simulink model "Droop_Control_MG_4DGs"  (R2024a)
settings: Solver=ode3  StartTime=0.0  StopTime=10  FixedStep=2e-5  RelTol=1e-3  EnableMultiTasking=on
InitFcn:
  | Kp_V = 4;
  | Ki_V = 800;
  | Kp_I = 5;
  | Ki_I = 110;
values from neighbouring files (symbols this model uses):
  DG = cell(1, numOfDGs)    [evaluateDesigns.m]
  Line = cell(1, numOfLines)    [evaluateDesigns.m]
  numOfDGs = size(B_il,1)    [OptimizeMGparameters.m]    (also in OptimizepValsMethod1.m; centralizedCodesign.m; centralizedCodesignFeasibility.m; centralizedLocalControlDesign-Mohammad’s Laptop.m)
  V_ref = 48    [Global_Controller_Synthesis.m]
undefined symbols (not defined in the file or in its folder): PlugIn, PlugOut, V_nom
libraries: spsSeriesRLCBranchLib x28, spsCurrentMeasurementLib x8, spsVoltageMeasurementLib x5, spsIdealSwitchLib x4, spsStairGeneratorLib x4, spsControlledCurrentSourceLib x4, spsDCVoltageSourceLib x4, spsDiodeLib x4, spsIGBTLib x4, simulink x4, spspowerguiLib x1
settings Model: Creator=Guo Fanghong Admin  LastModifiedBy=najaf
settings SolverCC: AlgebraicLoopSolver=TrustRegion
settings DataIOCC: LimitDataPoints=on  SaveFormat=Array  SignalLoggingSaveFormat=ModelDataLogs
settings OptimizationCC: ExpressionDepthLimit=2147483647  LifeSpan=inf
settings DebuggingCC: UnderspecifiedInitializationDetection=Classic  MergeDetectMultiDrivingBlocksExec=none  SolverPrmCheckMsg=warning  FcnCallInpInsideContextMsg=warning  UnconnectedInputMsg=warning  UnconnectedOutputMsg=warning  UnconnectedLineMsg=warning  StateNameClashWarn=warning  SFUnexpectedBacktrackingDiag=warning  SFNoUnconditionalDefaultTransitionDiag=warning  SFExecutionAtInitializationDiag=none  ArithmeticOperatorsInVariantConditions=warning
settings HardwareCC: ProdBitPerPointer=32  ProdBitPerSizeT=32  ProdBitPerPtrDiffT=32  ProdLargestAtomicFloat=None  ProdIntDivRoundTo=Undefined  ProdEndianess=Unspecified  ProdWordSize=32  ProdHWDeviceType=32-bit Generic
settings ModelReferenceCC: EnableRefExpFcnMdlSchedulingChecks=on  PropagateSignalLabelsOutOfModel=off
settings SFSimCC: SimUseLocalCustomCode=off  CustomCodeUndefinedFunction=UseInterfaceOnly
settings RTWCC: RTWUseLocalCustomCode=off  GPUComputeCapability=3.5
settings CodeAppCC: StateflowObjectComments=on
settings GRTTargetCC: TargetLangStandard=C89/C90 (ANSI)
settings ConfigComp: CovMetricSettings=dw  CovSaveCumulativeToWorkspaceVar=on  CovSaveSingleToWorkspaceVar=on  CovExternalEMLEnable=off  CovSFcnEnable=off
settings SimscapeCC: SimscapeNormalizeSystem=off

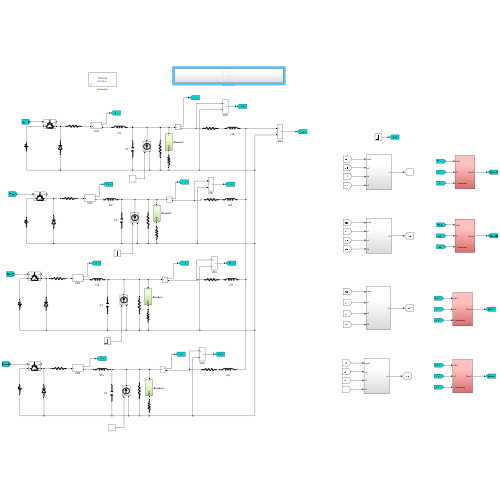
[thumbnail: Simulink's stored preview of the top-level diagram]
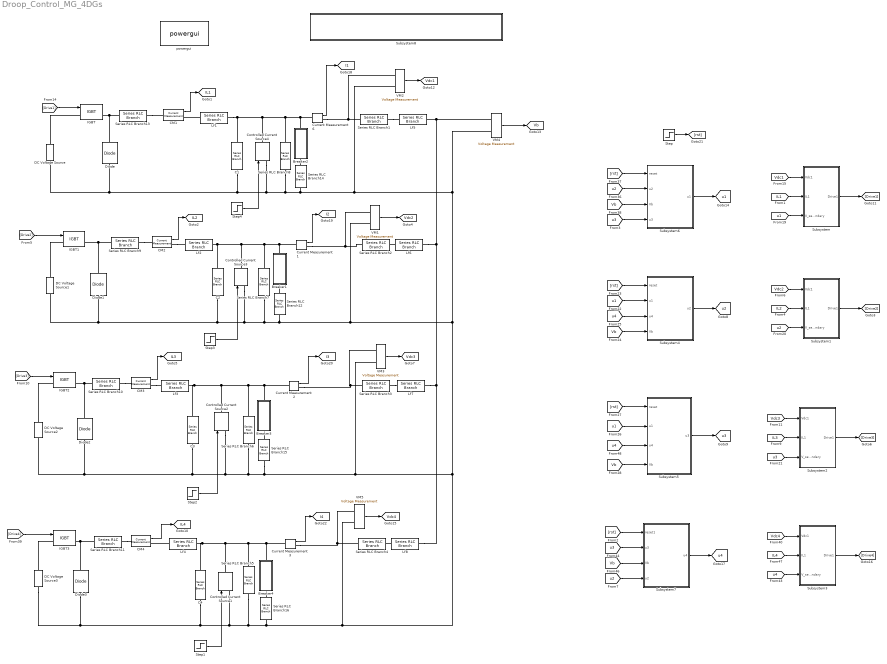
== system Droop_Control_MG_4DGs ==
  Breaker1 : Subsystem
  Breaker2 : Subsystem
  Breaker3 : Subsystem
  Breaker4 : Subsystem
  C1 : spsSeriesRLCBranchLib/Series RLC Branch  LConnTagsString=__new0  RConnTagsString=__new0  BranchType=C  Resistance=0  Inductance=0  SetiL0=off  InitialCurrent=0  Capacitance=DG{1}.C  Setx0=off  InitialVoltage=0  Measurements=None
  C2 : spsSeriesRLCBranchLib/Series RLC Branch  LConnTagsString=__new0  RConnTagsString=__new0  BranchType=C  Resistance=0  Inductance=0  SetiL0=off  InitialCurrent=0  Capacitance=DG{2}.C  Setx0=off  InitialVoltage=0  Measurements=None
  C3 : spsSeriesRLCBranchLib/Series RLC Branch  LConnTagsString=__new0  RConnTagsString=__new0  BranchType=C  Resistance=0  Inductance=0  SetiL0=off  InitialCurrent=0  Capacitance=DG{3}.C  Setx0=off  InitialVoltage=0  Measurements=None
  C4 : spsSeriesRLCBranchLib/Series RLC Branch  LConnTagsString=__new0  RConnTagsString=__new0  BranchType=C  Resistance=0  Inductance=0  SetiL0=off  InitialCurrent=0  Capacitance=DG{4}.C  Setx0=off  InitialVoltage=0  Measurements=None
  CM{1..4} (4 alike) : spsCurrentMeasurementLib/Current Measurement  PhasorSimulation=off  OutputType=Complex  PSBequivalent=0
  Controlled Current Source1 : spsControlledCurrentSourceLib/Controlled Current Source  Initialize=on  Source_Type=DC  Amplitude=5*DG{4}.IL  Phase=0  Frequency=0  Measurements=None
  Controlled Current Source2 : spsControlledCurrentSourceLib/Controlled Current Source  Initialize=on  Source_Type=DC  Amplitude=5*DG{3}.IL  Phase=0  Frequency=0  Measurements=None
  Controlled Current Source3 : spsControlledCurrentSourceLib/Controlled Current Source  Initialize=on  Source_Type=DC  Amplitude=5*DG{2}.IL  Phase=0  Frequency=0  Measurements=None
  Controlled Current Source4 : spsControlledCurrentSourceLib/Controlled Current Source  Initialize=on  Source_Type=DC  Amplitude=5*DG{1}.IL  Phase=0  Frequency=0  Measurements=None
  Current Measurement{1..3,6} (4 alike) : spsCurrentMeasurementLib/Current Measurement  PhasorSimulation=off  OutputType=Complex  PSBequivalent=0
  DC Voltage Source{,1..3} (4 alike) : spsDCVoltageSourceLib/DC Voltage Source  Amplitude=V_nom  Measurements=None
  Diode{,1..3} (4 alike) : spsDiodeLib/Diode  Ron=0.001  Lon=0  Vf=0.8  IC=0  UseSnubber=off  Rs=500  Cs=0  Measurements=off
  IGBT{,1..3} (4 alike) : spsIGBTLib/IGBT  Ron=0.001  Lon=0  Vf=1  Tf=1e-6  Tt=2e-6  IC=0  Rs=1e5  Cs=inf  Measurements=on
  Lf1 : spsSeriesRLCBranchLib/Series RLC Branch  LConnTagsString=__new0  RConnTagsString=__new0  BranchType=L  Resistance=0  Inductance=DG{1}.L  SetiL0=off  InitialCurrent=0  Capacitance=inf  Setx0=off  InitialVoltage=0  Measurements=Branch current
  Lf2 : spsSeriesRLCBranchLib/Series RLC Branch  LConnTagsString=__new0  RConnTagsString=__new0  BranchType=L  Resistance=0  Inductance=DG{2}.L  SetiL0=off  InitialCurrent=0  Capacitance=inf  Setx0=off  InitialVoltage=0  Measurements=Branch current
  Lf3 : spsSeriesRLCBranchLib/Series RLC Branch  LConnTagsString=__new0  RConnTagsString=__new0  BranchType=L  Resistance=0  Inductance=DG{3}.L  SetiL0=off  InitialCurrent=0  Capacitance=inf  Setx0=off  InitialVoltage=0  Measurements=Branch current
  Lf4 : spsSeriesRLCBranchLib/Series RLC Branch  LConnTagsString=__new0  RConnTagsString=__new0  BranchType=L  Resistance=0  Inductance=DG{4}.L  SetiL0=off  InitialCurrent=0  Capacitance=inf  Setx0=off  InitialVoltage=0  Measurements=Branch current
  Lf5 : spsSeriesRLCBranchLib/Series RLC Branch  LConnTagsString=__new0  RConnTagsString=__new0  BranchType=L  Resistance=0  Inductance=Line{1}.L  SetiL0=off  InitialCurrent=0  Capacitance=inf  Setx0=off  InitialVoltage=0  Measurements=Branch current
  Lf6 : spsSeriesRLCBranchLib/Series RLC Branch  LConnTagsString=__new0  RConnTagsString=__new0  BranchType=L  Resistance=0  Inductance=Line{2}.L  SetiL0=off  InitialCurrent=0  Capacitance=inf  Setx0=off  InitialVoltage=0  Measurements=Branch current
  Lf7 : spsSeriesRLCBranchLib/Series RLC Branch  LConnTagsString=__new0  RConnTagsString=__new0  BranchType=L  Resistance=0  Inductance=Line{3}.L  SetiL0=off  InitialCurrent=0  Capacitance=inf  Setx0=off  InitialVoltage=0  Measurements=Branch current
  Lf8 : spsSeriesRLCBranchLib/Series RLC Branch  LConnTagsString=__new0  RConnTagsString=__new0  BranchType=L  Resistance=0  Inductance=Line{4}.L  SetiL0=off  InitialCurrent=0  Capacitance=inf  Setx0=off  InitialVoltage=0  Measurements=Branch current
  Series RLC Branch1 : spsSeriesRLCBranchLib/Series RLC Branch  LConnTagsString=__new0  RConnTagsString=__new0  BranchType=R  Resistance=Line{1}.R  Inductance=0.25154  SetiL0=off  InitialCurrent=0  Capacitance=1e-6  Setx0=off  InitialVoltage=0  Measurements=None
  Series RLC Branch10 : spsSeriesRLCBranchLib/Series RLC Branch  LConnTagsString=__new0  RConnTagsString=__new0  BranchType=R  Resistance=DG{3}.R  Inductance=0.25154  SetiL0=off  InitialCurrent=0  Capacitance=1e-6  Setx0=off  InitialVoltage=0  Measurements=None
  Series RLC Branch11 : spsSeriesRLCBranchLib/Series RLC Branch  LConnTagsString=__new0  RConnTagsString=__new0  BranchType=R  Resistance=DG{4}.R  Inductance=0.25154  SetiL0=off  InitialCurrent=0  Capacitance=1e-6  Setx0=off  InitialVoltage=0  Measurements=None
  Series RLC Branch12 : spsSeriesRLCBranchLib/Series RLC Branch  LConnTagsString=__new0  RConnTagsString=__new0  BranchType=R  Resistance=0.5*DG{2}.Y  Inductance=1e-2  SetiL0=off  InitialCurrent=0  Capacitance=2.2e-3  Setx0=off  InitialVoltage=0  Measurements=None
  Series RLC Branch13 : spsSeriesRLCBranchLib/Series RLC Branch  LConnTagsString=__new0  RConnTagsString=__new0  BranchType=R  Resistance=DG{1}.R  Inductance=0.25154  SetiL0=off  InitialCurrent=0  Capacitance=1e-6  Setx0=off  InitialVoltage=0  Measurements=None
  Series RLC Branch14 : spsSeriesRLCBranchLib/Series RLC Branch  LConnTagsString=__new0  RConnTagsString=__new0  BranchType=R  Resistance=0.5*DG{1}.Y  Inductance=1e-2  SetiL0=off  InitialCurrent=0  Capacitance=2.2e-3  Setx0=off  InitialVoltage=0  Measurements=None
  Series RLC Branch15 : spsSeriesRLCBranchLib/Series RLC Branch  LConnTagsString=__new0  RConnTagsString=__new0  BranchType=R  Resistance=0.5*DG{3}.Y  Inductance=1e-2  SetiL0=off  InitialCurrent=0  Capacitance=2.2e-3  Setx0=off  InitialVoltage=0  Measurements=None
  Series RLC Branch16 : spsSeriesRLCBranchLib/Series RLC Branch  LConnTagsString=__new0  RConnTagsString=__new0  BranchType=R  Resistance=0.5*DG{4}.Y  Inductance=1e-2  SetiL0=off  InitialCurrent=0  Capacitance=2.2e-3  Setx0=off  InitialVoltage=0  Measurements=None
  Series RLC Branch2 : spsSeriesRLCBranchLib/Series RLC Branch  LConnTagsString=__new0  RConnTagsString=__new0  BranchType=R  Resistance=Line{2}.R  Inductance=0.25154  SetiL0=off  InitialCurrent=0  Capacitance=1e-6  Setx0=off  InitialVoltage=0  Measurements=None
  Series RLC Branch3 : spsSeriesRLCBranchLib/Series RLC Branch  LConnTagsString=__new0  RConnTagsString=__new0  BranchType=R  Resistance=Line{3}.R  Inductance=0.25154  SetiL0=off  InitialCurrent=0  Capacitance=1e-6  Setx0=off  InitialVoltage=0  Measurements=None
  Series RLC Branch4 : spsSeriesRLCBranchLib/Series RLC Branch  LConnTagsString=__new0  RConnTagsString=__new0  BranchType=R  Resistance=Line{4}.R  Inductance=0.25154  SetiL0=off  InitialCurrent=0  Capacitance=1e-6  Setx0=off  InitialVoltage=0  Measurements=None
  Series RLC Branch5 : spsSeriesRLCBranchLib/Series RLC Branch  LConnTagsString=__new0  RConnTagsString=__new0  BranchType=R  Resistance=DG{4}.Y  Inductance=0.25154  SetiL0=off  InitialCurrent=0  Capacitance=1e-6  Setx0=off  InitialVoltage=0  Measurements=None
  Series RLC Branch6 : spsSeriesRLCBranchLib/Series RLC Branch  LConnTagsString=__new0  RConnTagsString=__new0  BranchType=R  Resistance=DG{3}.Y  Inductance=0.25154  SetiL0=off  InitialCurrent=0  Capacitance=1e-6  Setx0=off  InitialVoltage=0  Measurements=None
  Series RLC Branch7 : spsSeriesRLCBranchLib/Series RLC Branch  LConnTagsString=__new0  RConnTagsString=__new0  BranchType=R  Resistance=DG{2}.Y  Inductance=0.25154  SetiL0=off  InitialCurrent=0  Capacitance=1e-6  Setx0=off  InitialVoltage=0  Measurements=None
  Series RLC Branch8 : spsSeriesRLCBranchLib/Series RLC Branch  LConnTagsString=__new0  RConnTagsString=__new0  BranchType=R  Resistance=DG{1}.Y  Inductance=0.25154  SetiL0=off  InitialCurrent=0  Capacitance=1e-6  Setx0=off  InitialVoltage=0  Measurements=None
  Series RLC Branch9 : spsSeriesRLCBranchLib/Series RLC Branch  LConnTagsString=__new0  RConnTagsString=__new0  BranchType=R  Resistance=DG{2}.R  Inductance=0.25154  SetiL0=off  InitialCurrent=0  Capacitance=1e-6  Setx0=off  InitialVoltage=0  Measurements=None
  Step : Step  SampleTime=0
  Step{1..4} (4 alike) : Step  Time=3  SampleTime=0
  Subsystem : Subsystem
  Subsystem1 : Subsystem
  Subsystem2 : Subsystem
  Subsystem3 : Subsystem
  Subsystem4 : Subsystem
  Subsystem5 : Subsystem
  Subsystem6 : Subsystem
  Subsystem7 : Subsystem
  Subsystem8 : Subsystem
  VM{1..5} (5 alike) : spsVoltageMeasurementLib/Voltage Measurement  PhasorSimulation=off  OutputType=Complex  PSBequivalent=0
  powergui : spspowerguiLib/powergui  Priority=1  SimulationMode=Discrete  SampleTime=2e-5  frequency=60  Iterations=50  frequencyindice=0  Pbase=100e6  ErrMax=1e-4  UnitsV=kV  UnitsW=MW  buscounter=0  FunctionMessages=off  echomessages=off  EnableUseOfTLC=off  CurrentSourceSwitches=off  DisableSnubberDevices=off  DisableRonSwitches=off  DisableVfSwitches=off  DisplayEquations=off  AutomaticDiscreteSolvers=off  SolverType=Tustin  Interpol=off  ExternalGateDelay=off  methode=off  Ts=0  x0status=steady  SPID=off  SwTol=0  HookPort=off  NonlinearTolerance=1e-4  nMaxIteration=100  ContinueOnMaxIteration=off  RestoreLinks=warning  ResistiveCurrentMeasurement=off  Frange=[0:2:500]  Ylog=off  Xlog=on  ShowGrid=off  save=off  variable=ZData  structure=0  ZoomFFT=off  StartTime=0.0  cycles=1  DisplayStyle=1  fundamental=60  FreqAxis=off  MaxFrequency=1000  frequencyindicesteady=1  RmsSteady=1  display=off
  tag scope: I1=global, I2=global, I3=global, I4=global, IL1=global, IL2=global, IL3=global, IL4=global, Vb=global, Vdc1=global, Vdc2=global, Vdc3=global, Vdc4=global, u1=global, u2=global, u3=global, u4=global
  wires:
  [Drive1] -> IGBT/1
  VM2/1 -> [Vdc1]
  CM1/1 -> [IL1]
  Subsystem/1(Drive1) -> [Drive1]
  [Vdc1] -> Subsystem/1(Vdc1)
  [IL1] -> Subsystem/2(IL1)
  [u1] -> Subsystem/3(V_secondary)
  [Drive2] -> IGBT1/1
  VM1/1 -> [Vdc2]
  CM2/1 -> [IL2]
  Subsystem1/1(Drive1) -> [Drive2]
  [Vdc2] -> Subsystem1/1(Vdc1)
  [IL2] -> Subsystem1/2(IL1)
  [u2] -> Subsystem1/3(V_secondary)
  [Drive3] -> IGBT2/1
  VM3/1 -> [Vdc3]
  CM3/1 -> [IL3]
  Subsystem2/1(Drive1) -> [Drive3]
  [Vdc3] -> Subsystem2/1(Vdc1)
  [IL3] -> Subsystem2/2(IL1)
  [u3] -> Subsystem2/3(V_secondary)
  Step/1 -> [rst]
  [u2] -> Subsystem6/2(u2)
  [rst] -> Subsystem6/1(reset)
  [Vb] -> Subsystem6/3(Vb)
  Subsystem6/1(u1) -> [u1]
  [u1] -> Subsystem4/2(u1)
  [rst] -> Subsystem4/1(reset)
  [Vb] -> Subsystem4/4(Vb)
  [u4] -> Subsystem4/3(u4)
  Subsystem4/1(u2) -> [u2]
  [u1] -> Subsystem5/2(u1)
  [rst] -> Subsystem5/1(reset)
  [Vb] -> Subsystem5/4(Vb)
  Subsystem5/1(u3) -> [u3]
  [Drive4] -> IGBT3/1
  VM5/1 -> [Vdc4]
  CM4/1 -> [IL4]
  Subsystem3/1(Drive1) -> [Drive4]
  [Vdc4] -> Subsystem3/1(Vdc1)
  [IL4] -> Subsystem3/2(IL1)
  [u4] -> Subsystem3/3(V_secondary)
  [u3] -> Subsystem7/2(u3)
  [rst] -> Subsystem7/1(reset1)
  [Vb] -> Subsystem7/3(Vb)
  Subsystem7/1(u4) -> [u4]
  [u4] -> Subsystem5/3(u4)
  VM4/1 -> [Vb]
  Step1/1 -> Controlled Current Source1/1
  Step2/1 -> Controlled Current Source2/1
  Step3/1 -> Controlled Current Source3/1
  Step4/1 -> Controlled Current Source4/1
  Current Measurement6/1 -> [I1]
  Current Measurement1/1 -> [I2]
  Current Measurement2/1 -> [I3]
  Current Measurement3/1 -> [I4]
  [u3] -> Subsystem6/4(u3)
  [u2] -> Subsystem7/4(u2)
  connections:
  C2/RConn1 -- Controlled Current Source3/LConn1 -- Series RLC Branch7/RConn1 -- Series RLC Branch12/RConn1 -- VM4/LConn2 -- VM2/LConn2 -- Series RLC Branch14/RConn1 -- Series RLC Branch8/RConn1 -- Controlled Current Source4/LConn1 -- C1/RConn1 -- Diode/LConn1 -- DC Voltage Source/LConn1 -- Controlled Current Source1/LConn1 -- Diode3/LConn1 -- DC Voltage Source3/LConn1 -- C4/RConn1 -- Series RLC Branch5/RConn1 -- Series RLC Branch16/RConn1 -- VM5/LConn2 -- Series RLC Branch15/RConn1 -- Series RLC Branch6/RConn1 -- Controlled Current Source2/LConn1 -- C3/RConn1 -- DC Voltage Source2/LConn1 -- Diode2/LConn1 -- VM3/LConn2 -- VM1/LConn2 -- Diode1/LConn1 -- DC Voltage Source1/LConn1
  Diode/RConn1 -- Series RLC Branch13/LConn1 -- IGBT/RConn1
  Lf1/RConn1 -- Current Measurement6/LConn1 -- Breaker2/RConn1 -- Series RLC Branch8/LConn1 -- Controlled Current Source4/RConn1 -- C1/LConn1
  IGBT/LConn1 -- DC Voltage Source/RConn1
  Diode1/RConn1 -- Series RLC Branch9/LConn1 -- IGBT1/RConn1
  IGBT1/LConn1 -- DC Voltage Source1/RConn1
  Series RLC Branch10/RConn1 -- CM3/LConn1
  IGBT2/LConn1 -- DC Voltage Source2/RConn1
  Series RLC Branch7/LConn1 -- Current Measurement1/LConn1 -- Breaker1/RConn1 -- Controlled Current Source3/RConn1 -- Lf2/RConn1 -- C2/LConn1
  Series RLC Branch6/LConn1 -- Current Measurement2/LConn1 -- Breaker3/RConn1 -- Controlled Current Source2/RConn1 -- Lf3/RConn1 -- C3/LConn1
  Lf8/RConn1 -- Lf7/RConn1 -- Lf6/RConn1 -- VM4/LConn1 -- Lf5/RConn1
  Series RLC Branch11/RConn1 -- CM4/LConn1
  Series RLC Branch4/LConn1 -- Current Measurement3/RConn1 -- VM5/LConn1
  IGBT3/LConn1 -- DC Voltage Source3/RConn1
  Lf1/LConn1 -- CM1/RConn1
  CM2/RConn1 -- Lf2/LConn1
  CM3/RConn1 -- Lf3/LConn1
  Lf4/LConn1 -- CM4/RConn1
  Series RLC Branch13/RConn1 -- CM1/LConn1
  Series RLC Branch9/RConn1 -- CM2/LConn1
  Diode2/RConn1 -- Series RLC Branch10/LConn1 -- IGBT2/RConn1
  Diode3/RConn1 -- Series RLC Branch11/LConn1 -- IGBT3/RConn1
  Series RLC Branch1/RConn1 -- Lf5/LConn1
  Series RLC Branch2/RConn1 -- Lf6/LConn1
  Series RLC Branch3/RConn1 -- Lf7/LConn1
  Series RLC Branch4/RConn1 -- Lf8/LConn1
  Series RLC Branch14/LConn1 -- Breaker2/LConn1
  Series RLC Branch12/LConn1 -- Breaker1/LConn1
  Series RLC Branch15/LConn1 -- Breaker3/LConn1
  Series RLC Branch16/LConn1 -- Breaker4/LConn1
  Series RLC Branch1/LConn1 -- VM2/LConn1 -- Current Measurement6/RConn1
  Series RLC Branch2/LConn1 -- Current Measurement1/RConn1 -- VM1/LConn1
  VM3/LConn1 -- Current Measurement2/RConn1 -- Series RLC Branch3/LConn1
  Controlled Current Source1/RConn1 -- Current Measurement3/LConn1 -- Breaker4/RConn1 -- Series RLC Branch5/LConn1 -- Lf4/RConn1 -- C4/LConn1

== system Droop_Control_MG_4DGs/Breaker1 ==
  Ideal Switch : spsIdealSwitchLib/Ideal Switch  Ron=0.001  Lon=0  IC=0  Rs=1e5  Cs=inf  Measurements=on
  Stair Generator : spsStairGeneratorLib/Stair Generator  t=[0,PlugOut,PlugIn]  e=[1, 0, 1]  Ts=0
  DG1 : PMIOPort  Side=Left
  + : PMIOPort  Port=2  Side=Right
  wires:
  Stair Generator/1 -> Ideal Switch/1
  connections:
  Ideal Switch/LConn1 -- DG1/RConn1
  Ideal Switch/RConn1 -- +/RConn1

== system Droop_Control_MG_4DGs/Breaker2 ==
  Ideal Switch : spsIdealSwitchLib/Ideal Switch  Ron=0.001  Lon=0  IC=0  Rs=1e5  Cs=inf  Measurements=on
  Stair Generator : spsStairGeneratorLib/Stair Generator  t=[0,PlugOut,PlugIn]  e=[1, 0, 1]  Ts=0
  DG1 : PMIOPort  Side=Left
  + : PMIOPort  Port=2  Side=Right
  wires:
  Stair Generator/1 -> Ideal Switch/1
  connections:
  Ideal Switch/RConn1 -- +/RConn1
  Ideal Switch/LConn1 -- DG1/RConn1

== system Droop_Control_MG_4DGs/Breaker3 ==
  Ideal Switch : spsIdealSwitchLib/Ideal Switch  Ron=0.001  Lon=0  IC=0  Rs=1e5  Cs=inf  Measurements=on
  Stair Generator : spsStairGeneratorLib/Stair Generator  t=[0,PlugOut,PlugIn]  e=[1, 0, 1]  Ts=0
  DG1 : PMIOPort  Side=Left
  + : PMIOPort  Port=2  Side=Right
  wires:
  Stair Generator/1 -> Ideal Switch/1
  connections:
  Ideal Switch/RConn1 -- +/RConn1
  Ideal Switch/LConn1 -- DG1/RConn1

== system Droop_Control_MG_4DGs/Breaker4 ==
  Ideal Switch : spsIdealSwitchLib/Ideal Switch  Ron=0.001  Lon=0  IC=0  Rs=1e5  Cs=inf  Measurements=on
  Stair Generator : spsStairGeneratorLib/Stair Generator  t=[0,PlugOut,PlugIn]  e=[1, 0, 1]  Ts=0
  DG1 : PMIOPort  Side=Left
  + : PMIOPort  Port=2  Side=Right
  wires:
  Stair Generator/1 -> Ideal Switch/1
  connections:
  Ideal Switch/LConn1 -- DG1/RConn1
  Ideal Switch/RConn1 -- +/RConn1

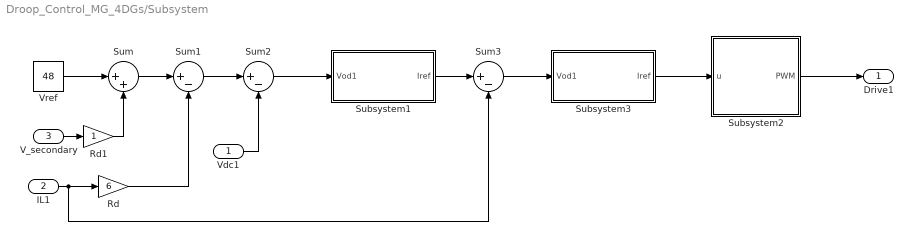
== system Droop_Control_MG_4DGs/Subsystem ==
  Vdc1 : Inport
  IL1 : Inport  Port=2
  V_secondary : Inport  Port=3
  Rd : Gain  Gain=6
  Rd1 : Gain
  Subsystem1 : Subsystem
      mask Display: disp('Voltage Controller')
  Subsystem2 : Subsystem
      mask Display: disp('PWM')
  Subsystem3 : Subsystem
      mask Display: disp('Current Controller')
  Sum : Sum  Inputs=|++
  Sum1 : Sum  Inputs=|+-
  Sum2 : Sum  Inputs=|+-
  Sum3 : Sum  Inputs=|+-
  Vref : Constant  Value=48
  Drive1 : Outport
  wires:
  Subsystem2/1(PWM) -> Drive1/1
  Vref/1 -> Sum/1
  Sum/1 -> Sum1/1
  V_secondary/1 -> Rd1/1
  Rd/1 -> Sum1/2
  IL1/1 -> Rd/1, Sum3/2
  Sum1/1 -> Sum2/1
  Vdc1/1 -> Sum2/2
  Sum2/1 -> Subsystem1/1(Vod1)
  Subsystem3/1(Iref) -> Subsystem2/1(u)
  Subsystem1/1(Iref) -> Sum3/1
  Sum3/1 -> Subsystem3/1(Vod1)
  Rd1/1 -> Sum/2

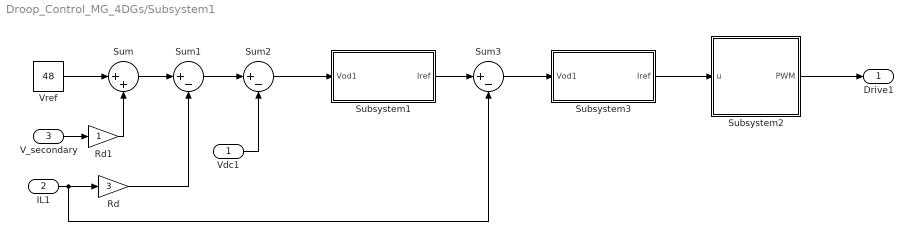
== system Droop_Control_MG_4DGs/Subsystem1 ==
  Vdc1 : Inport
  IL1 : Inport  Port=2
  V_secondary : Inport  Port=3
  Rd : Gain  Gain=3
  Rd1 : Gain
  Subsystem1 : Subsystem
      mask Display: disp('Voltage Controller')
  Subsystem2 : Subsystem
      mask Display: disp('PWM')
  Subsystem3 : Subsystem
      mask Display: disp('Current Controller')
  Sum : Sum  Inputs=|++
  Sum1 : Sum  Inputs=|+-
  Sum2 : Sum  Inputs=|+-
  Sum3 : Sum  Inputs=|+-
  Vref : Constant  Value=48
  Drive1 : Outport
  wires:
  Subsystem2/1(PWM) -> Drive1/1
  Vref/1 -> Sum/1
  Sum/1 -> Sum1/1
  V_secondary/1 -> Rd1/1
  Rd/1 -> Sum1/2
  IL1/1 -> Rd/1, Sum3/2
  Sum1/1 -> Sum2/1
  Vdc1/1 -> Sum2/2
  Sum2/1 -> Subsystem1/1(Vod1)
  Subsystem3/1(Iref) -> Subsystem2/1(u)
  Subsystem1/1(Iref) -> Sum3/1
  Sum3/1 -> Subsystem3/1(Vod1)
  Rd1/1 -> Sum/2

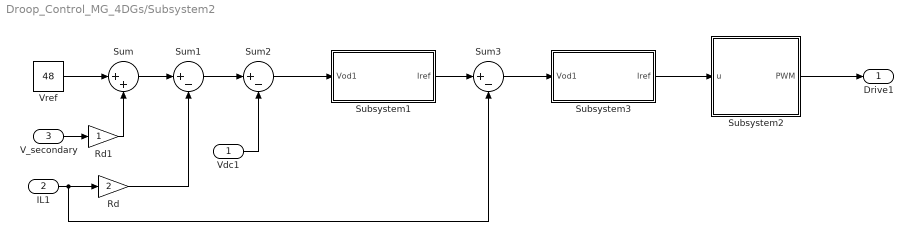
== system Droop_Control_MG_4DGs/Subsystem2 ==
  Vdc1 : Inport
  IL1 : Inport  Port=2
  V_secondary : Inport  Port=3
  Rd : Gain  Gain=2
  Rd1 : Gain
  Subsystem1 : Subsystem
      mask Display: disp('Voltage Controller')
  Subsystem2 : Subsystem
      mask Display: disp('PWM')
  Subsystem3 : Subsystem
      mask Display: disp('Current Controller')
  Sum : Sum  Inputs=|++
  Sum1 : Sum  Inputs=|+-
  Sum2 : Sum  Inputs=|+-
  Sum3 : Sum  Inputs=|+-
  Vref : Constant  Value=48
  Drive1 : Outport
  wires:
  Subsystem2/1(PWM) -> Drive1/1
  Vref/1 -> Sum/1
  Sum/1 -> Sum1/1
  V_secondary/1 -> Rd1/1
  Rd/1 -> Sum1/2
  IL1/1 -> Rd/1, Sum3/2
  Sum1/1 -> Sum2/1
  Vdc1/1 -> Sum2/2
  Sum2/1 -> Subsystem1/1(Vod1)
  Subsystem3/1(Iref) -> Subsystem2/1(u)
  Subsystem1/1(Iref) -> Sum3/1
  Sum3/1 -> Subsystem3/1(Vod1)
  Rd1/1 -> Sum/2

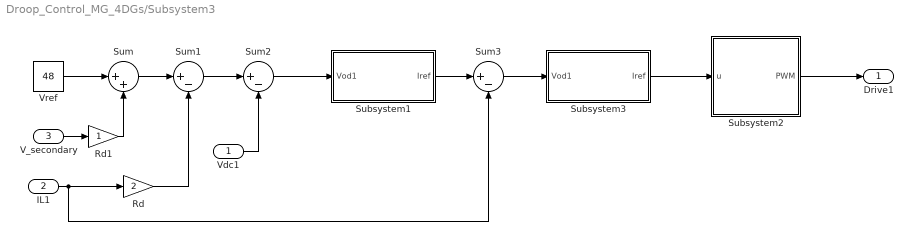
== system Droop_Control_MG_4DGs/Subsystem3 ==
  Vdc1 : Inport
  IL1 : Inport  Port=2
  V_secondary : Inport  Port=3
  Rd : Gain  Gain=2
  Rd1 : Gain
  Subsystem1 : Subsystem
      mask Display: disp('Voltage Controller')
  Subsystem2 : Subsystem
      mask Display: disp('PWM')
  Subsystem3 : Subsystem
      mask Display: disp('Current Controller')
  Sum : Sum  Inputs=|++
  Sum1 : Sum  Inputs=|+-
  Sum2 : Sum  Inputs=|+-
  Sum3 : Sum  Inputs=|+-
  Vref : Constant  Value=48
  Drive1 : Outport
  wires:
  Subsystem2/1(PWM) -> Drive1/1
  Vref/1 -> Sum/1
  Sum/1 -> Sum1/1
  V_secondary/1 -> Rd1/1
  Rd/1 -> Sum1/2
  IL1/1 -> Rd/1, Sum3/2
  Sum1/1 -> Sum2/1
  Vdc1/1 -> Sum2/2
  Sum2/1 -> Subsystem1/1(Vod1)
  Subsystem3/1(Iref) -> Subsystem2/1(u)
  Subsystem1/1(Iref) -> Sum3/1
  Sum3/1 -> Subsystem3/1(Vod1)
  Rd1/1 -> Sum/2

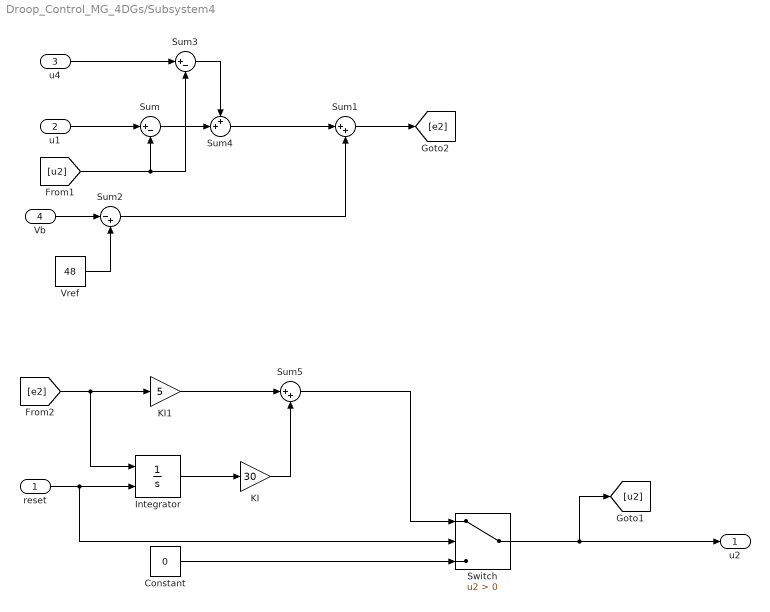
== system Droop_Control_MG_4DGs/Subsystem4 ==
  reset : Inport
  u1 : Inport  Port=2
  u4 : Inport  Port=3
  Vb : Inport  Port=4
  Constant : Constant  Value=0
  Integrator : Integrator  ExternalReset=rising
  KI : Gain  Gain=30
  KI1 : Gain  Gain=5
  Sum : Sum  Inputs=|+-
  Sum1 : Sum  Inputs=|++
  Sum2 : Sum  Inputs=|-+
  Sum3 : Sum  Inputs=|+-
  Sum4 : Sum  Inputs=++|
  Sum5 : Sum  Inputs=|++
  Switch : Switch  Criteria=u2 > Threshold  SaturateOnIntegerOverflow=off  InputSameDT=off
  Vref : Constant  Value=48
  u2 : Outport
  wires:
  Integrator/1 -> KI/1
  u1/1 -> Sum/1
  reset/1 -> Switch/2, Integrator/2
  Sum4/1 -> Sum1/1
  Vref/1 -> Sum2/2
  Vb/1 -> Sum2/1
  u4/1 -> Sum3/1
  Sum/1 -> Sum4/2
  Sum3/1 -> Sum4/1
  Constant/1 -> Switch/3
  Switch/1 -> [u2], u2/1
  Sum2/1 -> Sum1/2
  [u2] -> Sum3/2, Sum/2
  Sum1/1 -> [e2]
  [e2] -> Integrator/1, KI1/1
  KI1/1 -> Sum5/1
  KI/1 -> Sum5/2
  Sum5/1 -> Switch/1

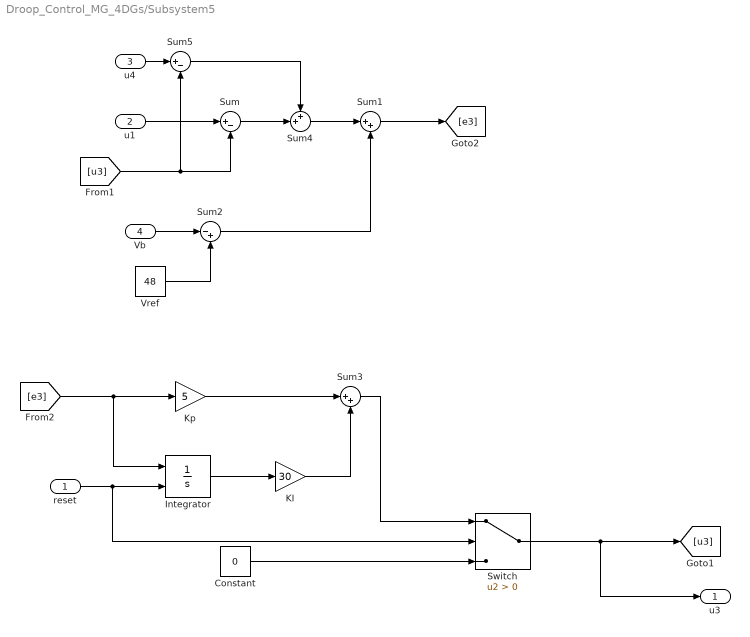
== system Droop_Control_MG_4DGs/Subsystem5 ==
  reset : Inport
  u1 : Inport  Port=2
  u4 : Inport  Port=3
  Vb : Inport  Port=4
  Constant : Constant  Value=0
  Integrator : Integrator  ExternalReset=rising
  KI : Gain  Gain=30
  Kp : Gain  Gain=5
  Sum : Sum  Inputs=|+-
  Sum1 : Sum  Inputs=|++
  Sum2 : Sum  Inputs=|-+
  Sum3 : Sum  Inputs=|++
  Sum4 : Sum  Inputs=++|
  Sum5 : Sum  Inputs=|+-
  Switch : Switch  Criteria=u2 > Threshold  SaturateOnIntegerOverflow=off  InputSameDT=off
  Vref : Constant  Value=48
  u3 : Outport
  wires:
  Integrator/1 -> KI/1
  u1/1 -> Sum/1
  Vref/1 -> Sum2/2
  Vb/1 -> Sum2/1
  reset/1 -> Switch/2, Integrator/2
  Constant/1 -> Switch/3
  Switch/1 -> u3/1, [u3]
  Sum2/1 -> Sum1/2
  [u3] -> Sum/2, Sum5/2
  Sum1/1 -> [e3]
  [e3] -> Integrator/1, Kp/1
  Kp/1 -> Sum3/1
  KI/1 -> Sum3/2
  Sum3/1 -> Switch/1
  u4/1 -> Sum5/1
  Sum/1 -> Sum4/2
  Sum5/1 -> Sum4/1
  Sum4/1 -> Sum1/1

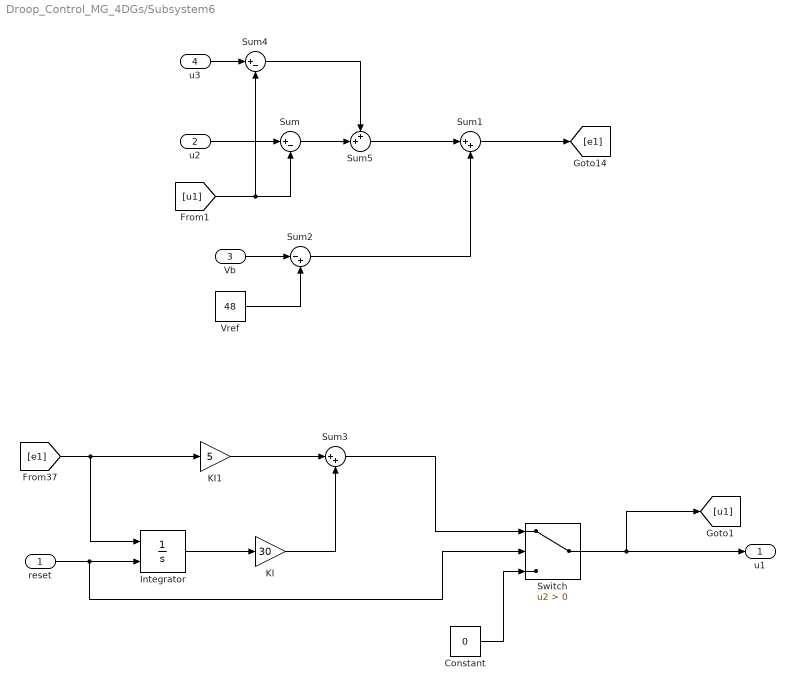
== system Droop_Control_MG_4DGs/Subsystem6 ==
  reset : Inport
  u2 : Inport  Port=2
  Vb : Inport  Port=3
  u3 : Inport  Port=4
  Constant : Constant  Value=0
  Integrator : Integrator  ExternalReset=rising
  KI : Gain  Gain=30
  KI1 : Gain  Gain=5
  Sum : Sum  Inputs=|+-
  Sum1 : Sum  Inputs=|++
  Sum2 : Sum  Inputs=|-+
  Sum3 : Sum  Inputs=|++
  Sum4 : Sum  Inputs=|+-
  Sum5 : Sum  Inputs=++|
  Switch : Switch  Criteria=u2 > Threshold  SaturateOnIntegerOverflow=off  InputSameDT=off
  Vref : Constant  Value=48
  u1 : Outport
  wires:
  Integrator/1 -> KI/1
  u2/1 -> Sum/1
  reset/1 -> Switch/2, Integrator/2
  Vref/1 -> Sum2/2
  Vb/1 -> Sum2/1
  Constant/1 -> Switch/3
  Switch/1 -> [u1], u1/1
  Sum1/1 -> [e1]
  Sum2/1 -> Sum1/2
  [e1] -> Integrator/1, KI1/1
  KI1/1 -> Sum3/1
  KI/1 -> Sum3/2
  Sum3/1 -> Switch/1
  [u1] -> Sum4/2, Sum/2
  u3/1 -> Sum4/1
  Sum/1 -> Sum5/2
  Sum4/1 -> Sum5/1
  Sum5/1 -> Sum1/1

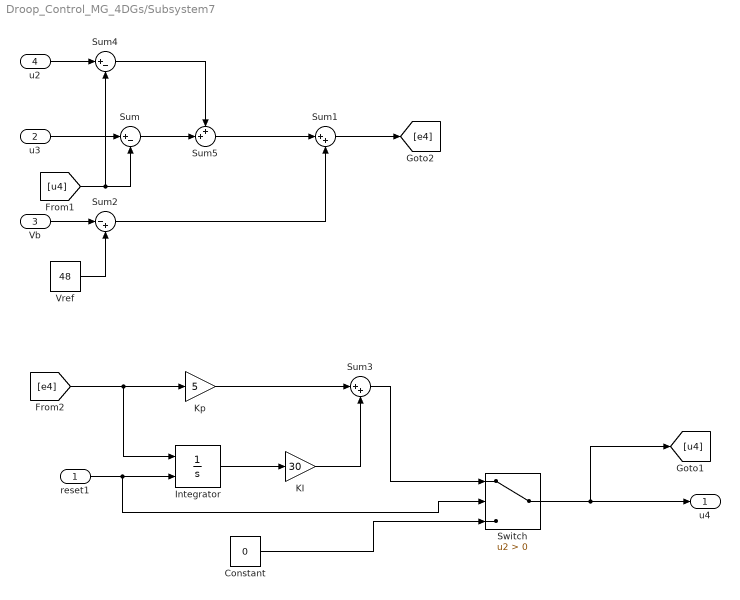
== system Droop_Control_MG_4DGs/Subsystem7 ==
  reset1 : Inport
  u3 : Inport  Port=2
  Vb : Inport  Port=3
  u2 : Inport  Port=4
  Constant : Constant  Value=0
  Integrator : Integrator  ExternalReset=rising
  KI : Gain  Gain=30
  Kp : Gain  Gain=5
  Sum : Sum  Inputs=|+-
  Sum1 : Sum  Inputs=|++
  Sum2 : Sum  Inputs=|-+
  Sum3 : Sum  Inputs=|++
  Sum4 : Sum  Inputs=|+-
  Sum5 : Sum  Inputs=++|
  Switch : Switch  Criteria=u2 > Threshold  SaturateOnIntegerOverflow=off  InputSameDT=off
  Vref : Constant  Value=48
  u4 : Outport
  wires:
  Integrator/1 -> KI/1
  u3/1 -> Sum/1
  Vref/1 -> Sum2/2
  Vb/1 -> Sum2/1
  reset1/1 -> Switch/2, Integrator/2
  Constant/1 -> Switch/3
  Switch/1 -> [u4], u4/1
  Sum2/1 -> Sum1/2
  Sum1/1 -> [e4]
  [e4] -> Integrator/1, Kp/1
  Kp/1 -> Sum3/1
  KI/1 -> Sum3/2
  Sum3/1 -> Switch/1
  [u4] -> Sum/2, Sum4/2
  u2/1 -> Sum4/1
  Sum/1 -> Sum5/2
  Sum4/1 -> Sum5/1
  Sum5/1 -> Sum1/1

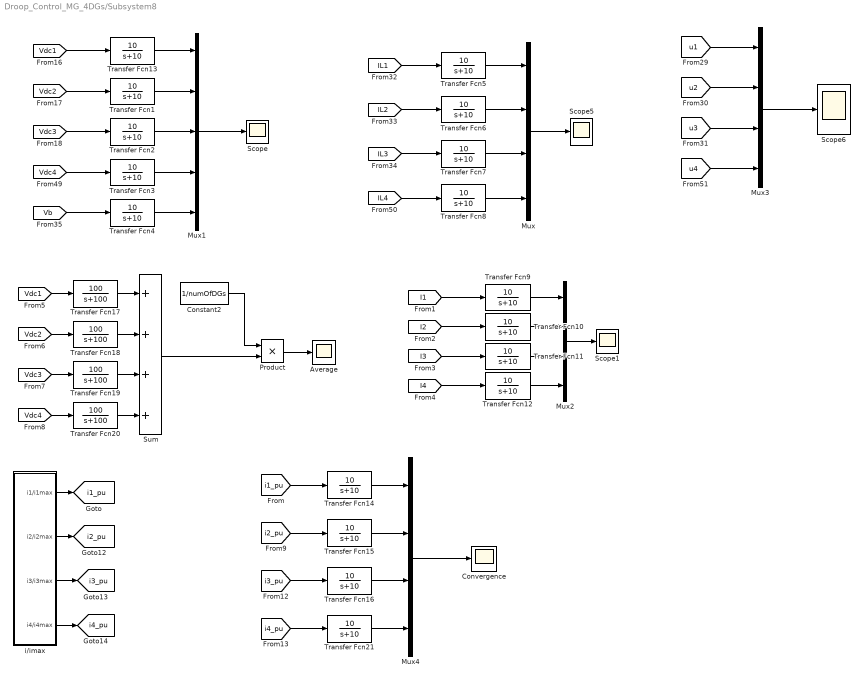
== system Droop_Control_MG_4DGs/Subsystem8 ==
  Average : Scope
  Constant2 : Constant  Value=1/numOfDGs
  Convergence : Scope
  Mux{,2..4} (4 alike) : Mux
  Mux1 : Mux  Inputs=5
  Product : Product
  Scope{,1,5..6} (4 alike) : Scope
  Sum : Sum  Inputs=++++
  Transfer Fcn{1..16,21} (17 alike) : TransferFcn  Numerator=[10]  Denominator=[1 10]
  Transfer Fcn{17..20} (4 alike) : TransferFcn  Numerator=[100]  Denominator=[1 100]
  i/imax : Subsystem
  tag scope: i1_pu=global, i2_pu=global, i3_pu=global, i4_pu=global
  wires:
  Mux/1 -> Scope5/1
  Mux3/1 -> Scope6/1
  Mux1/1 -> Scope/1
  [Vdc1] -> Transfer Fcn13/1
  [Vdc2] -> Transfer Fcn1/1
  [Vdc3] -> Transfer Fcn2/1
  [Vdc4] -> Transfer Fcn3/1
  [Vb] -> Transfer Fcn4/1
  [IL1] -> Transfer Fcn5/1
  [IL2] -> Transfer Fcn6/1
  [IL3] -> Transfer Fcn7/1
  [IL4] -> Transfer Fcn8/1
  [u1] -> Mux3/1
  [u2] -> Mux3/2
  [u3] -> Mux3/3
  [u4] -> Mux3/4
  Transfer Fcn13/1 -> Mux1/1
  Transfer Fcn1/1 -> Mux1/2
  Transfer Fcn2/1 -> Mux1/3
  Transfer Fcn3/1 -> Mux1/4
  Transfer Fcn4/1 -> Mux1/5
  Transfer Fcn5/1 -> Mux/1
  Transfer Fcn6/1 -> Mux/2
  Transfer Fcn7/1 -> Mux/3
  Transfer Fcn8/1 -> Mux/4
  Transfer Fcn20/1 -> Sum/4
  [Vdc2] -> Transfer Fcn18/1
  [Vdc3] -> Transfer Fcn19/1
  Transfer Fcn18/1 -> Sum/2
  [Vdc4] -> Transfer Fcn20/1
  [Vdc1] -> Transfer Fcn17/1
  Transfer Fcn19/1 -> Sum/3
  Product/1 -> Average/1
  Constant2/1 -> Product/1
  Sum/1 -> Product/2
  Transfer Fcn17/1 -> Sum/1
  Transfer Fcn9/1 -> Mux2/1
  Transfer Fcn12/1 -> Mux2/4
  Transfer Fcn11/1 -> Mux2/3
  Mux2/1 -> Scope1/1
  [I2] -> Transfer Fcn10/1
  [I1] -> Transfer Fcn9/1
  [I4] -> Transfer Fcn12/1
  [I3] -> Transfer Fcn11/1
  Transfer Fcn10/1 -> Mux2/2
  Transfer Fcn14/1 -> Mux4/1
  Transfer Fcn21/1 -> Mux4/4
  Transfer Fcn15/1 -> Mux4/2
  Transfer Fcn16/1 -> Mux4/3
  Mux4/1 -> Convergence/1
  [i4_pu] -> Transfer Fcn21/1
  i/imax/3(i3/i3max) -> [i3_pu]
  [i1_pu] -> Transfer Fcn14/1
  i/imax/2(i2/i2max) -> [i2_pu]
  i/imax/1(i1/i1max) -> [i1_pu]
  [i3_pu] -> Transfer Fcn16/1
  [i2_pu] -> Transfer Fcn15/1
  i/imax/4(i4/i4max) -> [i4_pu]

== system Droop_Control_MG_4DGs/Subsystem/Subsystem1 ==
  Vod1 : Inport
  Voltage Control : Subsystem
  Iref : Outport
  wires:
  Voltage Control/1(Out) -> Iref/1
  Vod1/1 -> Voltage Control/1(error)

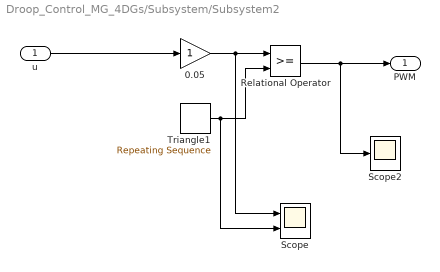
== system Droop_Control_MG_4DGs/Subsystem/Subsystem2 ==
  u : Inport
  0.05 : Gain
  Relational Operator : RelationalOperator  OutDataTypeStr=boolean  InputSameDT=off
  Scope : Scope  NumInputPorts=2
  Scope2 : Scope
  Triangle1 : simulink/Sources/Repeating Sequence  rep_seq_t=[0 40e-5 80e-5]  rep_seq_y=[0 1 0]
  PWM : Outport
  wires:
  0.05/1 -> Relational Operator/1, Scope/1
  Triangle1/1 -> Relational Operator/2, Scope/2
  u/1 -> 0.05/1
  Relational Operator/1 -> PWM/1, Scope2/1

== system Droop_Control_MG_4DGs/Subsystem/Subsystem3 ==
  Vod1 : Inport
  Current Control : Subsystem
  Iref : Outport
  wires:
  Current Control/1(Out) -> Iref/1
  Vod1/1 -> Current Control/1(Error)

== system Droop_Control_MG_4DGs/Subsystem1/Subsystem1 ==
  Vod1 : Inport
  Voltage Control : Subsystem
  Iref : Outport
  wires:
  Voltage Control/1(Out) -> Iref/1
  Vod1/1 -> Voltage Control/1(error)

== system Droop_Control_MG_4DGs/Subsystem1/Subsystem2 ==
  u : Inport
  0.05 : Gain
  Relational Operator : RelationalOperator  OutDataTypeStr=boolean  InputSameDT=off
  Scope : Scope  NumInputPorts=2
  Scope2 : Scope
  Triangle1 : simulink/Sources/Repeating Sequence  rep_seq_t=[0 40e-5 80e-5]  rep_seq_y=[0 1 0]
  PWM : Outport
  wires:
  0.05/1 -> Relational Operator/1, Scope/1
  Triangle1/1 -> Relational Operator/2, Scope/2
  u/1 -> 0.05/1
  Relational Operator/1 -> PWM/1, Scope2/1

== system Droop_Control_MG_4DGs/Subsystem1/Subsystem3 ==
  Vod1 : Inport
  Current Control : Subsystem
  Iref : Outport
  wires:
  Current Control/1(Out) -> Iref/1
  Vod1/1 -> Current Control/1(Error)

== system Droop_Control_MG_4DGs/Subsystem2/Subsystem1 ==
  Vod1 : Inport
  Voltage Control : Subsystem
  Iref : Outport
  wires:
  Voltage Control/1(Out) -> Iref/1
  Vod1/1 -> Voltage Control/1(error)

== system Droop_Control_MG_4DGs/Subsystem2/Subsystem2 ==
  u : Inport
  0.05 : Gain
  Relational Operator : RelationalOperator  OutDataTypeStr=boolean  InputSameDT=off
  Scope : Scope  NumInputPorts=2
  Scope2 : Scope
  Triangle1 : simulink/Sources/Repeating Sequence  rep_seq_t=[0 40e-5 80e-5]  rep_seq_y=[0 1 0]
  PWM : Outport
  wires:
  0.05/1 -> Relational Operator/1, Scope/1
  Triangle1/1 -> Relational Operator/2, Scope/2
  u/1 -> 0.05/1
  Relational Operator/1 -> PWM/1, Scope2/1

== system Droop_Control_MG_4DGs/Subsystem2/Subsystem3 ==
  Vod1 : Inport
  Current Control : Subsystem
  Iref : Outport
  wires:
  Current Control/1(Out) -> Iref/1
  Vod1/1 -> Current Control/1(Error)

== system Droop_Control_MG_4DGs/Subsystem3/Subsystem1 ==
  Vod1 : Inport
  Voltage Control : Subsystem
  Iref : Outport
  wires:
  Voltage Control/1(Out) -> Iref/1
  Vod1/1 -> Voltage Control/1(error)

== system Droop_Control_MG_4DGs/Subsystem3/Subsystem2 ==
  u : Inport
  0.05 : Gain
  Relational Operator : RelationalOperator  OutDataTypeStr=boolean  InputSameDT=off
  Scope : Scope  NumInputPorts=2
  Scope2 : Scope
  Triangle1 : simulink/Sources/Repeating Sequence  rep_seq_t=[0 40e-5 80e-5]  rep_seq_y=[0 1 0]
  PWM : Outport
  wires:
  0.05/1 -> Relational Operator/1, Scope/1
  Triangle1/1 -> Relational Operator/2, Scope/2
  u/1 -> 0.05/1
  Relational Operator/1 -> PWM/1, Scope2/1

== system Droop_Control_MG_4DGs/Subsystem3/Subsystem3 ==
  Vod1 : Inport
  Current Control : Subsystem
  Iref : Outport
  wires:
  Current Control/1(Out) -> Iref/1
  Vod1/1 -> Current Control/1(Error)

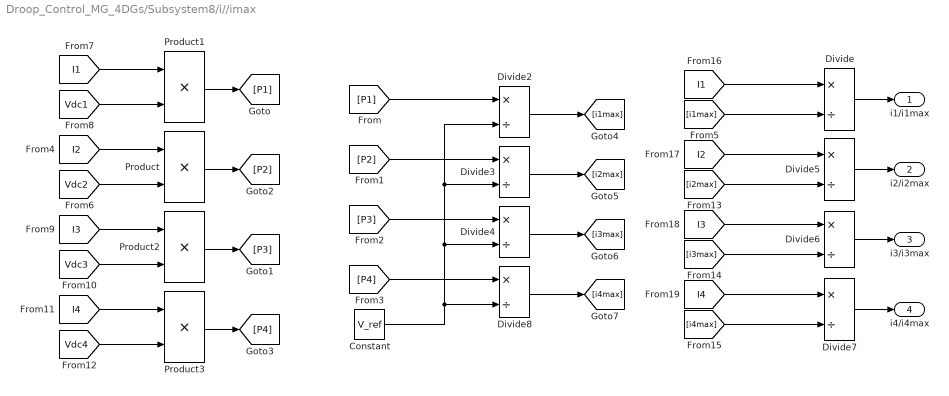
== system Droop_Control_MG_4DGs/Subsystem8/i//imax ==
  Constant : Constant  Value=V_ref
  Divide{,2..8} (8 alike) : Product  Inputs=*/
  Product{,1..3} (4 alike) : Product
  i1/i1max : Outport  VectorParamsAs1DForOutWhenUnconnected=off
  i2/i2max : Outport  Port=2  VectorParamsAs1DForOutWhenUnconnected=off
  i3/i3max : Outport  Port=3  VectorParamsAs1DForOutWhenUnconnected=off
  i4/i4max : Outport  Port=4  VectorParamsAs1DForOutWhenUnconnected=off
  wires:
  Divide/1 -> i1/i1max/1
  Divide5/1 -> i2/i2max/1
  Divide6/1 -> i3/i3max/1
  Divide7/1 -> i4/i4max/1
  [Vdc3] -> Product2/2
  [Vdc1] -> Product1/2
  [Vdc2] -> Product/2
  [I1] -> Product1/1
  [I2] -> Product/1
  [Vdc4] -> Product3/2
  [I4] -> Product3/1
  [I3] -> Product2/1
  Product1/1 -> [P1]
  Product2/1 -> [P3]
  Product/1 -> [P2]
  Product3/1 -> [P4]
  [P1] -> Divide2/1
  [P2] -> Divide3/1
  [P3] -> Divide4/1
  [P4] -> Divide8/1
  Constant/1 -> Divide8/2, Divide4/2, Divide3/2, Divide2/2
  Divide8/1 -> [i4max]
  Divide4/1 -> [i3max]
  Divide3/1 -> [i2max]
  Divide2/1 -> [i1max]
  [i1max] -> Divide/2
  [i2max] -> Divide5/2
  [i3max] -> Divide6/2
  [i4max] -> Divide7/2
  [I1] -> Divide/1
  [I2] -> Divide5/1
  [I3] -> Divide6/1
  [I4] -> Divide7/1

== system Droop_Control_MG_4DGs/Subsystem/Subsystem1/Voltage Control ==
  error : Inport
  Add2 : Sum
  Integrator : Integrator
  Kp4 : Gain  Gain=Kp_V  SaturateOnIntegerOverflow=on  OutDataTypeStr=Inherit: Same as input  ParamDataTypeStr=Inherit: Same as input
  Kp5 : Gain  Gain=Ki_V  SaturateOnIntegerOverflow=on  OutDataTypeStr=Inherit: Same as input  ParamDataTypeStr=Inherit: Same as input
  Saturation1 : Saturate  UpperLimit=10000  LowerLimit=-10000
  Out : Outport
  wires:
  Kp5/1 -> Add2/2
  Saturation1/1 -> Out/1
  error/1 -> Integrator/1, Kp4/1
  Kp4/1 -> Add2/1
  Add2/1 -> Saturation1/1
  Integrator/1 -> Kp5/1

== system Droop_Control_MG_4DGs/Subsystem/Subsystem3/Current Control ==
  Error : Inport
  Add2 : Sum
  Integrator : Integrator
  Kp4 : Gain  Gain=Kp_I  SaturateOnIntegerOverflow=on  OutDataTypeStr=Inherit: Same as input  ParamDataTypeStr=Inherit: Same as input
  Kp5 : Gain  Gain=Ki_I  SaturateOnIntegerOverflow=on  OutDataTypeStr=Inherit: Same as input  ParamDataTypeStr=Inherit: Same as input
  Saturation1 : Saturate  UpperLimit=10000  LowerLimit=-10000
  Out : Outport
  wires:
  Kp5/1 -> Add2/2
  Saturation1/1 -> Out/1
  Kp4/1 -> Add2/1
  Add2/1 -> Saturation1/1
  Integrator/1 -> Kp5/1
  Error/1 -> Kp4/1, Integrator/1

== system Droop_Control_MG_4DGs/Subsystem1/Subsystem1/Voltage Control ==
  error : Inport
  Add2 : Sum
  Integrator : Integrator
  Kp4 : Gain  Gain=Kp_V  SaturateOnIntegerOverflow=on  OutDataTypeStr=Inherit: Same as input  ParamDataTypeStr=Inherit: Same as input
  Kp5 : Gain  Gain=Ki_V  SaturateOnIntegerOverflow=on  OutDataTypeStr=Inherit: Same as input  ParamDataTypeStr=Inherit: Same as input
  Saturation1 : Saturate  UpperLimit=10000  LowerLimit=-10000
  Out : Outport
  wires:
  Kp5/1 -> Add2/2
  Saturation1/1 -> Out/1
  error/1 -> Integrator/1, Kp4/1
  Kp4/1 -> Add2/1
  Add2/1 -> Saturation1/1
  Integrator/1 -> Kp5/1

== system Droop_Control_MG_4DGs/Subsystem1/Subsystem3/Current Control ==
  Error : Inport
  Add2 : Sum
  Integrator : Integrator
  Kp4 : Gain  Gain=Kp_I  SaturateOnIntegerOverflow=on  OutDataTypeStr=Inherit: Same as input  ParamDataTypeStr=Inherit: Same as input
  Kp5 : Gain  Gain=Ki_I  SaturateOnIntegerOverflow=on  OutDataTypeStr=Inherit: Same as input  ParamDataTypeStr=Inherit: Same as input
  Saturation1 : Saturate  UpperLimit=10000  LowerLimit=-10000
  Out : Outport
  wires:
  Kp5/1 -> Add2/2
  Saturation1/1 -> Out/1
  Kp4/1 -> Add2/1
  Add2/1 -> Saturation1/1
  Integrator/1 -> Kp5/1
  Error/1 -> Kp4/1, Integrator/1

== system Droop_Control_MG_4DGs/Subsystem2/Subsystem1/Voltage Control ==
  error : Inport
  Add2 : Sum
  Integrator : Integrator
  Kp4 : Gain  Gain=Kp_V  SaturateOnIntegerOverflow=on  OutDataTypeStr=Inherit: Same as input  ParamDataTypeStr=Inherit: Same as input
  Kp5 : Gain  Gain=Ki_V  SaturateOnIntegerOverflow=on  OutDataTypeStr=Inherit: Same as input  ParamDataTypeStr=Inherit: Same as input
  Saturation1 : Saturate  UpperLimit=10000  LowerLimit=-10000
  Out : Outport
  wires:
  Kp5/1 -> Add2/2
  Saturation1/1 -> Out/1
  error/1 -> Integrator/1, Kp4/1
  Kp4/1 -> Add2/1
  Add2/1 -> Saturation1/1
  Integrator/1 -> Kp5/1

== system Droop_Control_MG_4DGs/Subsystem2/Subsystem3/Current Control ==
  Error : Inport
  Add2 : Sum
  Integrator : Integrator
  Kp4 : Gain  Gain=Kp_I  SaturateOnIntegerOverflow=on  OutDataTypeStr=Inherit: Same as input  ParamDataTypeStr=Inherit: Same as input
  Kp5 : Gain  Gain=Ki_I  SaturateOnIntegerOverflow=on  OutDataTypeStr=Inherit: Same as input  ParamDataTypeStr=Inherit: Same as input
  Saturation1 : Saturate  UpperLimit=10000  LowerLimit=-10000
  Out : Outport
  wires:
  Kp5/1 -> Add2/2
  Saturation1/1 -> Out/1
  Kp4/1 -> Add2/1
  Add2/1 -> Saturation1/1
  Integrator/1 -> Kp5/1
  Error/1 -> Kp4/1, Integrator/1

== system Droop_Control_MG_4DGs/Subsystem3/Subsystem1/Voltage Control ==
  error : Inport
  Add2 : Sum
  Integrator : Integrator
  Kp4 : Gain  Gain=Kp_V  SaturateOnIntegerOverflow=on  OutDataTypeStr=Inherit: Same as input  ParamDataTypeStr=Inherit: Same as input
  Kp5 : Gain  Gain=Ki_V  SaturateOnIntegerOverflow=on  OutDataTypeStr=Inherit: Same as input  ParamDataTypeStr=Inherit: Same as input
  Saturation1 : Saturate  UpperLimit=10000  LowerLimit=-10000
  Out : Outport
  wires:
  Kp5/1 -> Add2/2
  Saturation1/1 -> Out/1
  error/1 -> Integrator/1, Kp4/1
  Kp4/1 -> Add2/1
  Add2/1 -> Saturation1/1
  Integrator/1 -> Kp5/1

== system Droop_Control_MG_4DGs/Subsystem3/Subsystem3/Current Control ==
  Error : Inport
  Add2 : Sum
  Integrator : Integrator
  Kp4 : Gain  Gain=Kp_I  SaturateOnIntegerOverflow=on  OutDataTypeStr=Inherit: Same as input  ParamDataTypeStr=Inherit: Same as input
  Kp5 : Gain  Gain=Ki_I  SaturateOnIntegerOverflow=on  OutDataTypeStr=Inherit: Same as input  ParamDataTypeStr=Inherit: Same as input
  Saturation1 : Saturate  UpperLimit=10000  LowerLimit=-10000
  Out : Outport
  wires:
  Kp5/1 -> Add2/2
  Saturation1/1 -> Out/1
  Kp4/1 -> Add2/1
  Add2/1 -> Saturation1/1
  Integrator/1 -> Kp5/1
  Error/1 -> Kp4/1, Integrator/1
